simulink library "pmm"  (R2021b)
settings: Solver=VariableStepAuto  StartTime=0.0  StopTime=10.0  RelTol=1e-3
undefined symbols (not defined in the file or in its folder): APMM_CoolgFanActCurr_X_pct, APMM_EWP1Curr_X_c, APMM_EWP3Curr_X_c, APMM_LVBattChktime_X_enum, APMM_LVBattChrgtime_X_enum, APMM_LVChrgLv_X_mV, ENUM_ANTITHEFT_ALARM, ENUM_ANTITHEFT_ARM, ENUM_ANTITHEFT_DISARM, ENUM_ANTITHEFT_WAIT, ENUM_APSSYSTEMSTA_REMOTEACTIVE, ENUM_CHRGPLUGSTA_NONE, ENUM_CRASHSTATE_FRONTFIRSTLV, ENUM_CRASHSTATE_LEFTSIDE, ENUM_CRASHSTATE_RIGHTSIDE, ENUM_DRIVETRAIN_AWD, ENUM_DRIVETRAIN_FWD, ENUM_DRIVETRAIN_RWD, ENUM_GEARACTUALPOSN_D, ENUM_GEARACTUALPOSN_N, ENUM_GEARACTUALPOSN_R, ENUM_HVBATTREADYPRE_READY, ENUM_OTACHKSTA_NOREQUEST, ENUM_OTACHKSTA_NOTIMEOUT, ENUM_OTACHKSTA_TIMEOUT, ENUM_PDKEYRAWLULOCK_INLOCK, ENUM_PDKEYRAWLULOCK_INUNLOCK, ENUM_PDKEYRAWPS_INPS, ENUM_PDKEYSTA_LOCK, ENUM_PDKEYSTA_PS, ENUM_PDKEYSTA_UNAVALIABLE, ENUM_PDKEYSTA_UNLOCK, ENUM_POWERSTA_OFF, ENUM_POWERSTA_OFFC, ENUM_POWERSTA_STANDBY, ENUM_PWRREQOTA_NOREQUEST, ENUM_PWRREQOTA_REQPOWEROFF, ENUM_PWRREQOTA_REQPOWERSTDBY, ENUM_PWRSTASW_READY, ENUM_V2LSTA_NOPLUG, ENUM_VEHICLETYPE_D31L24, FALSE, KPMM_AllDoorClosedHoldTime_s, KPMM_APSAllowThd_pct, KPMM_BattDownFailtime_s, KPMM_BattUpFailtime_s, KPMM_BattUpResetRty_cnt, KPMM_BattUpResetSW_flg, KPMM_BattUpResetTO_s, KPMM_BattUpRstDlyTO_s, KPMM_BrakeSWHoldTime_s, KPMM_ChrgPlugHoldTime_s, KPMM_DCDCDisableFailtime_s, KPMM_DCDCEnableFailtime_s, KPMM_DCDCVSET_V, KPMM_DCDCVSETLVChrg_V, KPMM_DoorSWHoldTime_s, KPMM_DriverSafetyChkFailtime_s, KPMM_DrivetrainSelect_enum_ovrdflg, KPMM_DrivetrainSelect_enum_ovrdval ... (+61)
libraries: simulink x29, hcu_lib x17
(part 4 of 6)

== system pmm/PMM/PMM/PMM_State_Machine/OFF_C.LVBattChrgTimeCal ==
  SilentChrgLv : Inport
  f : TriggerPort  TriggerType=function-call  VariantControl=(inherit)
      settings: CopyFcn=Stateflow.SLINSF.SimulinkMan.removeBlockPreDeleteFcn  PreDeleteFcn=Stateflow.SLINSF.SimulinkMan.unsafePredeleteFcn
  MPMM_LVBattChrgtime_Y_s : Lookup_n-D  NumberOfTableDimensions=1  BreakpointsForDimension1=APMM_LVBattChrgtime_X_enum  Table=MPMM_LVBattChrgtime_Y_s  ExtrapMethod=Clip  InternalRulePriority=Speed  RndMeth=Simplest  InputSameDT=on
  LVBattChrgTime : Outport
  wires:
  MPMM_LVBattChrgtime_Y_s/1 -> LVBattChrgTime/1  "VPMM_LVBattChrgtimeOut_s"
  SilentChrgLv/1 -> MPMM_LVBattChrgtime_Y_s/1

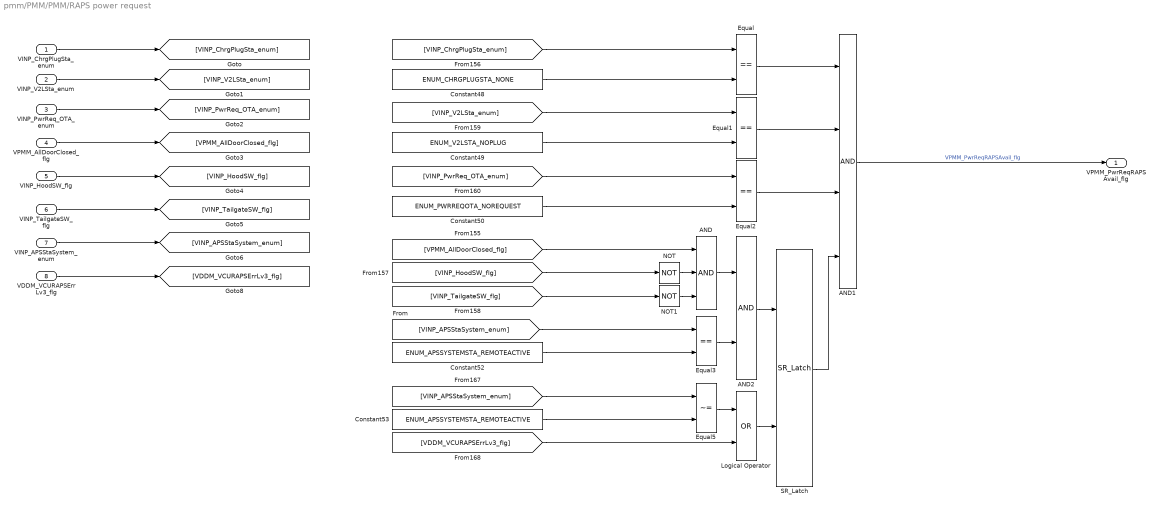
== system pmm/PMM/PMM/RAPS power request ==
  VINP_ChrgPlugSta_enum : Inport
  VINP_V2LSta_enum : Inport  Port=2
  VINP_PwrReq_OTA_enum : Inport  Port=3
  VPMM_AllDoorClosed_flg : Inport  Port=4
  VINP_HoodSW_flg : Inport  Port=5
  VINP_TailgateSW_flg : Inport  Port=6
  VINP_APSStaSystem_enum : Inport  Port=7
  VDDM_VCURAPSErrLv3_flg : Inport  Port=8
  AND : Logic  Inputs=3  AllPortsSameDT=off  OutDataTypeStr=boolean
  AND1 : Logic  Inputs=4  AllPortsSameDT=off  OutDataTypeStr=boolean
  AND2 : Logic  AllPortsSameDT=off  OutDataTypeStr=boolean
  Constant48 : Constant  Value=ENUM_CHRGPLUGSTA_NONE
  Constant49 : Constant  Value=ENUM_V2LSTA_NOPLUG
  Constant50 : Constant  Value=ENUM_PWRREQOTA_NOREQUEST
  Constant52 : Constant  Value=ENUM_APSSYSTEMSTA_REMOTEACTIVE
  Constant53 : Constant  Value=ENUM_APSSYSTEMSTA_REMOTEACTIVE
  Equal{,1..3} (4 alike) : RelationalOperator  Operator===  OutDataTypeStr=boolean  RndMeth=Simplest
  Equal5 : RelationalOperator  Operator=~=  OutDataTypeStr=boolean  RndMeth=Simplest
  Logical Operator : Logic  Operator=OR  AllPortsSameDT=off  OutDataTypeStr=boolean
  NOT : Logic  Operator=NOT  AllPortsSameDT=off  OutDataTypeStr=boolean
  NOT1 : Logic  Operator=NOT  AllPortsSameDT=off  OutDataTypeStr=boolean
  SR_Latch : hcu_lib/Basic_Blocks/SR_Latch
  VPMM_PwrReqRAPSAvail_flg : Outport
  wires:
  Equal3/1 -> AND2/2
  [VPMM_AllDoorClosed_flg] -> AND/1
  Constant52/1 -> Equal3/2
  Constant50/1 -> Equal2/2
  NOT1/1 -> AND/3
  Constant53/1 -> Equal5/2
  AND1/1 -> VPMM_PwrReqRAPSAvail_flg/1  "VPMM_PwrReqRAPSAvail_flg"
  Constant48/1 -> Equal/2
  Equal5/1 -> Logical Operator/1
  [VINP_PwrReq_OTA_enum] -> Equal2/1
  [VINP_ChrgPlugSta_enum] -> Equal/1
  [VINP_TailgateSW_flg] -> NOT1/1
  Constant49/1 -> Equal1/2
  AND/1 -> AND2/1
  [VINP_V2LSta_enum] -> Equal1/1
  [VINP_APSStaSystem_enum] -> Equal5/1
  Equal/1 -> AND1/1
  [VINP_HoodSW_flg] -> NOT/1
  NOT/1 -> AND/2
  Equal2/1 -> AND1/3
  [VINP_APSStaSystem_enum] -> Equal3/1
  AND2/1 -> SR_Latch/1
  Equal1/1 -> AND1/2
  SR_Latch/1 -> AND1/4
  VINP_ChrgPlugSta_enum/1 -> [VINP_ChrgPlugSta_enum]
  VINP_V2LSta_enum/1 -> [VINP_V2LSta_enum]
  VINP_PwrReq_OTA_enum/1 -> [VINP_PwrReq_OTA_enum]
  VPMM_AllDoorClosed_flg/1 -> [VPMM_AllDoorClosed_flg]
  VINP_HoodSW_flg/1 -> [VINP_HoodSW_flg]
  VINP_TailgateSW_flg/1 -> [VINP_TailgateSW_flg]
  VINP_APSStaSystem_enum/1 -> [VINP_APSStaSystem_enum]
  [VDDM_VCURAPSErrLv3_flg] -> Logical Operator/2
  Logical Operator/1 -> SR_Latch/2
  VDDM_VCURAPSErrLv3_flg/1 -> [VDDM_VCURAPSErrLv3_flg]

== stateflow chart pmm/PMM/PMM/RequirementManagementForPowerUp ==
  state RequirementManagementForPowerUp
    (default) -> (junction 135)
    RequirementManagementForPowerUp -> (junction 135) [order 2]
    (junction 135) -> (junction 3) : {VPMM_PwrUpReq_enum = ENUM_PWRUPREQ_NOREQUEST;
        |  VPMM_PwrStaSelect_enum = ENUM_PWRSTASELECT_NOREQUEST;}
    (junction 3) -> (junction 158) [order 1] : [(VPMM_PowerSta_enum == ENUM_POWERSTA_OFF || ...
        |   VPMM_PowerSta_enum == ENUM_POWERSTA_STANDBY) && ...
        |  VPMM_OTAPwrReqOFFChkSta_enum != ENUM_OTACHKSTA_NOTIMEOUT && ...
        |  VPMM_OTAPwrReqStdChkSta_enum != ENUM_OTACHKSTA_NOTIMEOUT]
    (junction 158) -> (junction 5) [order 1] : [(VPMM_DetectDoorOpened_flg || ...
        |   VPMM_BrkPedalRisingEdge_flg || ...
        |   (VPMM_BrkPedalPressed_flg && VPMM_PreOFF_flg) || ...
        |   (VPMM_DetectDoorOpened_flg && VPMM_PreOFF_flg)) && ...
        |  VPMM_PowerSta_enum == ENUM_POWERSTA_STANDBY]
        | {VPMM_PwrStaSelect_enum = ENUM_PWRSTASELECT_GOON;}
    (junction 3) -> (junction 6) [order 2]
    (junction 158) -> (junction 7) [order 2]
    (junction 5) -> (junction 8)
    (junction 7) -> (junction 235) [order 1] : [VPMM_ChrgPlugInRisingEdge_flg && ...
        |  VPMM_PowerSta_enum == ENUM_POWERSTA_STANDBY]
        | {VPMM_PwrStaSelect_enum = ENUM_PWRSTASELECT_GOOFFC;}
    (junction 8) -> (junction 167) [order 1] : [VPMM_PowerUpState_enum == ENUM_PUSTATE_POWERUPFAIL]
    (junction 7) -> (junction 162) [order 2]
    (junction 235) -> (junction 173)
    (junction 8) -> (junction 169) [order 2] : {VPMM_PwrUpReq_enum = ENUM_PWRUPREQ_USERREQPU;}
    (junction 167) -> (junction 171)
    (junction 162) -> (junction 164) [order 1] : [VPMM_LVSilentChrgReqStd_flg || VPMM_LVSilentChrgReq_flg || ...
        |  (VINP_EvccAplusPwrUpReq_flg && VINP_ChrgPlugSta_enum != ENUM_CHRGPLUGSTA_NONE)]
        | {VPMM_PwrStaSelect_enum = ENUM_PWRSTASELECT_GOOFFC;}
    (junction 164) -> (junction 173) [order 1] : [VTQD_GearActualPosn_enum == ENUM_GEARACTUALPOSN_P && ...
        |  VINP_VehSpeed_kph < 2 && ...
        |  !VINP_HoodSW_flg]
    (junction 162) -> (junction 237) [order 2]
    (junction 164) -> (junction 225) [order 2]
    (junction 173) -> (junction 239)
    (junction 237) -> (junction 239) [order 1] : [(VINP_PwrReq_OTA_enum == ENUM_PWRREQOTA_REQPOWERON && VINP_HVBattSOC_pct > KPMM_HVBattSOCPwrDwnThd_pct) || ...
        | (VINP_APSPwrReq_enum == ENUM_PWRREQPAPS_REQPWRREADY && VPMM_PwrReqRAPSAvail_flg)]
        | {VPMM_PwrStaSelect_enum = ENUM_PWRSTASELECT_GOON;}
    (junction 237) -> (junction 242) [order 2]
    (junction 239) -> (junction 244)
    (junction 242) -> (junction 244) [order 1] : [(VINP_SchedChgwake_flg == ENUM_SCHEDCHG_WAKE && ...
        |   VINP_ChrgPlugSta_enum != ENUM_CHRGPLUGSTA_NONE)]
        | {VPMM_PwrStaSelect_enum = ENUM_PWRSTASELECT_GOOFFC;}
    (junction 242) -> (junction 248) [order 2]
    (junction 244) -> (junction 250)
    (junction 248) -> (junction 250) [order 1] : [VINP_HVBPreheatPrecoolSta_enum == ENUM_HVBPRESTA_PREHEAT || ...
        |  VINP_HVBPreheatPrecoolSta_enum == ENUM_HVBPRESTA_PRECOOL]
        | {VPMM_PwrStaSelect_enum = ENUM_PWRSTASELECT_GOOFFA;}
    (junction 248) -> (junction 179) [order 2]
    (junction 250) -> (junction 194)
    (junction 179) -> (junction 181) [order 1] : [VINP_RePwrReqTbox_enum == ENUM_REPWRREQTBOX_REQVEHCHK || ...
        |  VINP_RePwrReqTbox_enum == ENUM_REPWRREQTBOX_REQDTC || ...
        |  VINP_RePwrReqTbox_enum == ENUM_REPWRREQTBOX_REQRADIO || ...
        |  VINP_RePwrReqTbox_enum == ENUM_REPWRREQTBOX_REQON || ...
        |  VINP_RePwrReqDKCT_enum == ENUM_REPWRREQDKC_REQVEHCHK || ...
        |  VINP_RePwrReqDKCT_enum == ENUM_REPWRREQDKC_REQDTC || ...
        |  VINP_RePwrReqDKCT_enum == ENUM_REPWRREQDKC_REQRADIO || ...
        |  VINP_RePwrReqDKCT_enum == ENUM_REPWRREQDKC_REQON]
        | {VPMM_PwrStaSelect_enum = ENUM_PWRSTASELECT_GOON;}
    (junction 179) -> (junction 183) [order 2]
    (junction 181) -> (junction 185)
    (junction 183) -> (junction 185) [order 1] : [VINP_RePwrReqTbox_enum == ENUM_REPWRREQTBOX_REQACTEMP || ...
        |  VINP_RePwrReqDKCT_enum == ENUM_REPWRREQDKC_REQACTEMP]
        | {VPMM_PwrStaSelect_enum = ENUM_PWRSTASELECT_GOOFFA;}
    (junction 183) -> (junction 190) [order 2]
    (junction 185) -> (junction 9)
    (junction 9) -> (junction 194) [order 1] : [VTQD_GearActualPosn_enum == ENUM_GEARACTUALPOSN_P && ...
        |  !VPMM_BMSWarn_flg && ...
        |  VINP_VehSpeed_kph < 2 && ...
        |  VINP_HVBattSOC_pct > KPMM_HVBattSOCPwrDwnThd_pct && ...
        |  VPMM_AllDoorClosed_flg && ...
        |  !VINP_HoodSW_flg && ...
        |  !VINP_TailgateSW_flg && ...
        |  VBCM_AntitheftSta_enum == ENUM_ANTITHEFT_ARM]
        | {VPMM_ReVehThdChkSta_enum = ENUM_REVEHSTA_CHECKOK;}
    (junction 194) -> (junction 197) [order 1] : [VPMM_PowerUpState_enum == ENUM_PUSTATE_POWERUPFAIL]
    (junction 9) -> (junction 11) [order 2]
    (junction 194) -> (junction 204) [order 2] : {VPMM_PwrUpReq_enum = ENUM_PWRUPREQ_SYSREQPU;}
    (junction 197) -> (junction 200)
    (junction 11) -> (junction 12) [order 1] : [VTQD_GearActualPosn_enum != ENUM_GEARACTUALPOSN_P]
        | {VPMM_ReVehThdChkSta_enum = ENUM_REVEHSTA_GEARPOSITIONERROR;}
    (junction 11) -> (junction 15) [order 2]
    (junction 15) -> (junction 16) [order 1] : [VPMM_BMSWarn_flg]
        | {VPMM_ReVehThdChkSta_enum = ENUM_REVEHSTA_HVBERR;}
    (junction 15) -> (junction 17) [order 2]
    (junction 17) -> (junction 18) [order 1] : [VINP_VehSpeed_kph >= 2]
        | {VPMM_ReVehThdChkSta_enum = ENUM_REVEHSTA_VEHNOTSTEADYSTATE;}
    (junction 17) -> (junction 21) [order 2]
    (junction 21) -> (junction 22) [order 1] : [VBCM_AntitheftSta_enum != ENUM_ANTITHEFT_ARM]
        | {VPMM_ReVehThdChkSta_enum = ENUM_REVEHSTA_ANTITHEFTNOTARM;}
    (junction 21) -> (junction 26) [order 2]
    (junction 26) -> (junction 27) [order 1] : [!VPMM_AllDoorClosed_flg || ...
        |  VINP_HoodSW_flg || ...
        |  VINP_TailgateSW_flg]
        | {VPMM_ReVehThdChkSta_enum = ENUM_REVEHSTA_ANYDOOROPEN;}
    (junction 26) -> (junction 29) [order 2]
    (junction 29) -> (junction 30) [order 1] : [VINP_HVBattSOC_pct <= KPMM_HVBattSOCPwrDwnThd_pct]
        | {VPMM_ReVehThdChkSta_enum = ENUM_REVEHSTA_HVBSOCLOW;}
    (junction 29) -> (junction 31) [order 2] : {VPMM_ReVehThdChkSta_enum = ENUM_REVEHSTA_CHECKINVALID;}
    (junction 169) -> (junction 204)
    (junction 204) -> (junction 32)
    RequirementManagementForPowerUp -> (junction 32) [order 1] : [VPMM_PwrUpChk_flg]
        | {VPMM_PwrUpChk_flg = FALSE;}
    (junction 32) -> (junction 139) [order 1] : [VPMM_PowerUpState_enum == ENUM_PUSTATE_COMPLETED]
        | {VPMM_PwrUpChkFailtimer_s = 0;}
    (junction 32) -> (junction 141) [order 2]
    (junction 141) -> (junction 143) [order 1] : [VPMM_PwrUpChkFailtimer_s >= KPMM_PwrUpChkFailtime_s]
        | {VPMM_PwrUpChkFailtimer_s = 0;}
    (junction 141) -> (junction 145) [order 2] : {VPMM_PwrUpChk_flg = TRUE;
        |  VPMM_PwrUpChkFailtimer_s += task_time_s;}
  data: task_time_s input; VINP_HVBPreheatPrecoolSta_enum input; VINP_HVBattSOC_pct input; VINP_HoodSW_flg input; VINP_TailgateSW_flg input; VINP_SchedChgwake_flg input; VINP_VehSpeed_kph input; VPMM_AllDoorClosed_flg input; VBCM_AntitheftSta_enum input; VPMM_BMSWarn_flg input; VPMM_BrkPedalPressed_flg input; VPMM_BrkPedalRisingEdge_flg input; VPMM_ChrgPlugInRisingEdge_flg input; VPMM_DetectDoorOpened_flg input; VPMM_LVSilentChrgReq_flg input boolean; VPMM_PowerSta_enum input uint8; VTQD_GearActualPosn_enum input; VINP_PwrReq_OTA_enum input; VINP_RePwrReqDKCT_enum input; VINP_RePwrReqTbox_enum input; VPMM_PwrStaSelect_enum output; VPMM_PwrUpReq_enum output; VPMM_ReVehThdChkSta_enum output; ENUM_ANTITHEFT_ARM parameter; ENUM_GEARACTUALPOSN_P parameter; ENUM_HVBPRESTA_PRECOOL parameter; ENUM_HVBPRESTA_PREHEAT parameter; ENUM_POWERSTA_OFF parameter; ENUM_POWERSTA_STANDBY parameter; ENUM_PWRREQOTA_REQPOWERON parameter; ENUM_PWRSTASELECT_GOOFFA parameter; ENUM_PWRSTASELECT_GOOFFC parameter; ENUM_PWRSTASELECT_GOON parameter; ENUM_PWRSTASELECT_NOREQUEST parameter; ENUM_PWRUPREQ_NOREQUEST parameter; ENUM_PWRUPREQ_SYSREQPU parameter; ENUM_PWRUPREQ_USERREQPU parameter; ENUM_REPWRREQDKC_REQACTEMP parameter; ENUM_REPWRREQDKC_REQDTC parameter; ENUM_REPWRREQDKC_REQON parameter; ENUM_REPWRREQDKC_REQRADIO parameter; ENUM_REPWRREQDKC_REQVEHCHK parameter; ENUM_REPWRREQTBOX_REQACTEMP parameter; ENUM_REPWRREQTBOX_REQDTC parameter; ENUM_REPWRREQTBOX_REQON parameter; ENUM_REPWRREQTBOX_REQRADIO parameter; ENUM_REPWRREQTBOX_REQVEHCHK parameter; ENUM_REVEHSTA_ANTITHEFTNOTARM parameter; ENUM_REVEHSTA_ANYDOOROPEN parameter; ENUM_REVEHSTA_CHECKINVALID parameter; ENUM_REVEHSTA_CHECKOK parameter; ENUM_REVEHSTA_GEARPOSITIONERROR parameter; ENUM_REVEHSTA_HVBERR parameter; ENUM_REVEHSTA_HVBSOCLOW parameter; ENUM_REVEHSTA_VEHNOTSTEADYSTATE parameter; ENUM_SCHEDCHG_WAKE parameter; KPMM_PwrUpChkFailtime_s parameter; VPMM_PowerUpState_enum input uint8; VPMM_PwrUpChkFailtimer_s local single; VPMM_PwrUpChk_flg local boolean; ENUM_PUSTATE_COMPLETED parameter; FALSE parameter; TRUE parameter; VINP_ChrgPlugSta_enum input uint8; VINP_EvccAplusPwrUpReq_flg input boolean; VPMM_LVSilentChrgReqStd_flg input boolean; ENUM_PUSTATE_POWERUPFAIL parameter; VPMM_PreOFF_flg input boolean; ENUM_CHRGPLUGSTA_NONE parameter; VPMM_OTAPwrReqOFFChkSta_enum input uint8; VPMM_OTAPwrReqStdChkSta_enum input uint8; ENUM_OTACHKSTA_NOTIMEOUT parameter; KPMM_HVBattSOCPwrDwnThd_pct input; VINP_APSPwrReq_enum input uint8; VPMM_PwrReqRAPSAvail_flg input boolean; ENUM_PWRREQPAPS_REQPWRREADY parameter

== stateflow chart pmm/PMM/PMM/RequirementManagementForPowerStateConstrain ==
  state RequirementManagementForPowerStateConstrain
    (default) -> (junction 2) : {VPMM_TCountSta_enum = ENUM_TCOUNTSTA_NOCOUNTING;
        |  VPMM_PwrOffTimer_s = 0;}
    RequirementManagementForPowerStateConstrain -> (junction 2) [order 2]
    (junction 2) -> (junction 3) : {VPMM_PwrStaConstraint_enum = ENUM_PWRCONSTRAINT_NOREQUEST;}
    RequirementManagementForPowerStateConstrain -> (junction 3) [order 1] : [VPMM_ConstraintLoop_flg]
        | {VPMM_ConstraintLoop_flg = FALSE;}
    (junction 3) -> (junction 4) [order 1] : [VPMM_PowerSta_enum == ENUM_POWERSTA_ON || ...
        |  VPMM_PowerSta_enum == ENUM_POWERSTA_OFFA || ...
        |  VPMM_PowerSta_enum == ENUM_POWERSTA_OFFC]
    (junction 4) -> (junction 5) [order 1] : [VINP_PwrReq_OTA_enum == ENUM_PWRREQOTA_REQPOWERON || ...
        |  VINP_OFFACMODE_enum == ENUM_OFFACMODE_CAMP]
    (junction 3) -> (junction 6) [order 2]
    (junction 4) -> (junction 7) [order 2]
    (junction 5) -> (junction 8) : {VPMM_PwrStaConstraint_enum = ENUM_PWRCONSTRAINT_PWRSTAON;}
    (junction 7) -> (junction 8) [order 1] : [VINP_AVMOFFRecButt_flg == ENUM_AVMOFFRECBUTT_ON || ...
        |  VINP_OFFACMODE_enum == ENUM_OFFACMODE_PET || ...
        |  VINP_OFFACMODE_enum == ENUM_OFFACMODE_ON || ...
        |  VINP_HVBPreheatPrecoolSta_enum == ENUM_HVBPRESTA_PREHEAT || ...
        |  VINP_HVBPreheatPrecoolSta_enum == ENUM_HVBPRESTA_PRECOOL]
        | {VPMM_PwrStaConstraint_enum = ENUM_PWRCONSTRAINT_HVACTIVE;}
    (junction 7) -> (junction 80) [order 2]
    (junction 8) -> (junction 9) : {VPMM_TCountSta_enum = ENUM_TCOUNTSTA_NOCOUNTING;
        |  VPMM_PwrOffTimer_s = 0;
        |  VPMM_ConstraintLoop_flg = TRUE;}
    (junction 80) -> (junction 82) [order 1] : [VPMM_TCountSta_enum == ENUM_TCOUNTSTA_COUNTINGFINISH]
    (junction 82) -> (junction 90) [order 1] : [VPMM_PwrStaSW_enum == ENUM_PWRSTASW_PWRDOWN]
    (junction 80) -> (junction 10) [order 2]
    (junction 82) -> (junction 84) [order 2]
    (junction 90) -> (junction 92) : {VPMM_TCountSta_enum = ENUM_TCOUNTSTA_NOCOUNTING;}
    (junction 10) -> (junction 11) [order 1] : [(VPMM_PowerOffTSet_s > 0 && ...
        |   (VINP_RePwrReqTbox_enum == ENUM_REPWRREQTBOX_REQVEHCHK || ...
        |    VINP_RePwrReqTbox_enum == ENUM_REPWRREQTBOX_REQDTC || ...
        |    VINP_RePwrReqTbox_enum == ENUM_REPWRREQTBOX_REQRADIO || ...
        |    VINP_RePwrReqTbox_enum == ENUM_REPWRREQTBOX_REQON)) || ...
        |  (VPMM_PowerOffTSetDKC_enum > 0 && ...
        |   (VINP_RePwrReqDKCT_enum == ENUM_REPWRREQDKC_REQVEHCHK || ...
        |    VINP_RePwrReqDKCT_enum == ENUM_REPWRREQDKC_REQDTC || ...
        |    VINP_RePwrReqDKCT_enum == ENUM_REPWRREQDKC_REQRADIO || ...
        |    VINP_RePwrReqDKCT_enum == ENUM_REPWRREQDKC_REQON))]
    (junction 10) -> (junction 12) [order 2]
    (junction 11) -> (junction 13) : {VPMM_PwrStaConstraint_enum = ENUM_PWRCONSTRAINT_ONFORTIME;}
    (junction 12) -> (junction 13) [order 1] : [(VPMM_PowerOffTSet_s > 0 && ...
        |   VINP_RePwrReqTbox_enum == ENUM_REPWRREQTBOX_REQACTEMP) || ...
        |  (VPMM_PowerOffTSetDKC_enum > 0 && ...
        |   VINP_RePwrReqDKCT_enum == ENUM_REPWRREQDKC_REQACTEMP)]
        | {VPMM_PwrStaConstraint_enum = ENUM_PWRCONSTRAINT_HVFORTIME;}
    (junction 13) -> (junction 14) [order 1] : [(VPMM_PowerOffTSet_s >= VPMM_PowerOffTSetDKC_enum && VPMM_PwrOffTimer_s >= VPMM_PowerOffTSet_s) || ...
        |  (VPMM_PowerOffTSetDKC_enum > VPMM_PowerOffTSet_s && VPMM_PwrOffTimer_s >= VPMM_PowerOffTSetDKC_enum)]
    (junction 12) -> (junction 15) [order 2] : {VPMM_TCountSta_enum = ENUM_TCOUNTSTA_NOCOUNTING;
        |  VPMM_PwrOffTimer_s = 0;}
    (junction 13) -> (junction 16) [order 2] : {VPMM_TCountSta_enum = ENUM_TCOUNTSTA_TIMMERCOUNTING;
        |  VPMM_PwrOffTimer_s += task_time_s;
        |  VPMM_ConstraintLoop_flg = TRUE;}
    (junction 14) -> (junction 17) : {VPMM_TCountSta_enum = ENUM_TCOUNTSTA_COUNTINGFINISH;
        |  VPMM_PwrStaConstraint_enum = ENUM_PWRCONSTRAINT_NOREQUEST;
        |  VPMM_PwrOffTimer_s = 0;}
  data: task_time_s input; VPMM_PowerSta_enum input; VINP_AVMOFFRecButt_flg input; VINP_HVBPreheatPrecoolSta_enum input; VINP_OFFACMODE_enum input; VPMM_PowerOffTSet_s input; VPMM_PowerOffTSetDKC_enum input; VINP_PwrReq_OTA_enum input; VINP_RePwrReqDKCT_enum input; VINP_RePwrReqTbox_enum input; VPMM_PwrStaConstraint_enum output; VPMM_TCountSta_enum output; VPMM_PwrOffTimer_s local single; ENUM_AVMOFFRECBUTT_ON parameter; ENUM_HVBPRESTA_PRECOOL parameter; ENUM_HVBPRESTA_PREHEAT parameter; ENUM_OFFACMODE_CAMP parameter; ENUM_OFFACMODE_ON parameter; ENUM_OFFACMODE_PET parameter; ENUM_POWERSTA_OFFA parameter; ENUM_POWERSTA_OFFC parameter; ENUM_POWERSTA_ON parameter; ENUM_PWRCONSTRAINT_HVACTIVE parameter; ENUM_PWRCONSTRAINT_HVFORTIME parameter; ENUM_PWRCONSTRAINT_NOREQUEST parameter; ENUM_PWRCONSTRAINT_ONFORTIME parameter; ENUM_PWRCONSTRAINT_PWRSTAON parameter; ENUM_PWRREQOTA_REQPOWERON parameter; ENUM_REPWRREQDKC_REQACTEMP parameter; ENUM_REPWRREQDKC_REQDTC parameter; ENUM_REPWRREQDKC_REQON parameter; ENUM_REPWRREQDKC_REQRADIO parameter; ENUM_REPWRREQDKC_REQVEHCHK parameter; ENUM_REPWRREQTBOX_REQACTEMP parameter; ENUM_REPWRREQTBOX_REQDTC parameter; ENUM_REPWRREQTBOX_REQON parameter; ENUM_REPWRREQTBOX_REQRADIO parameter; ENUM_REPWRREQTBOX_REQVEHCHK parameter; ENUM_TCOUNTSTA_COUNTINGFINISH parameter; ENUM_TCOUNTSTA_NOCOUNTING parameter; ENUM_TCOUNTSTA_TIMMERCOUNTING parameter; VPMM_ConstraintLoop_flg local boolean; FALSE parameter; TRUE parameter; VPMM_PwrStaSW_enum input; ENUM_PWRSTASW_PWRDOWN parameter
